simulink model "Linearization"  (R2022a)
settings: Solver=VariableStepAuto  StartTime=0.0  StopTime=100  RelTol=1e-3
undefined symbols (not defined in the file): Aactuator, ac, AeroCoeff, ControlAllocation, DUmax, DUmin, EngineTable, F, fcs, ft, g, hground, IC, kg, LandingGear, Light, LPmethod, m, MIL, Mode_deflection_aileron, Mode_deflection_elevator, Mode_deflection_rudder, Mode_deflection_TVC_y, Mode_deflection_TVC_z, N, Ninv_2nozzle, Ninv_no_nozzle, PIController, s, Sensor, slug, state0, sysID_DAQ, sysID_OBES, Umax_2nozzle, Umax_no_nozzle, Umin_2nozzle, Umin_no_nozzle, WMM2020
libraries: aerolibconvert2 x19, slpidlib x6, simulink x6, sharedutil x4, aerolibatmos2 x3, aerolibwind2 x3, aerolibbdyn x3, aerolibgravity2 x2, sharedtransform x1
(part 7 of 9)

== system Linearization/pqr NDI Controller/control matrix g1/Yawing  ==
  note: 註：因為 $\delta$ 單位是度(degree)，所以需要額外用 ${\left(\frac{\pi }{180°}\right)}$ 做單位換算
  note: $g_{r_{\delta_{rz} } } =\frac{-I_x l_T }{I_x I_z -I_{xz}^2 }\frac{T}{2}∙{\left(\frac{\pi }{180°}\right)}$
  note: 有指定port dimensions=[1,9]
  note: 1  gp_dra1
      | 2  gp_dla1
      | 3  gp_dre1
      | 4  gp_dle1
      | 5  gp_dr1
      | 6  gp_dra2
      | 7  gp_dla2
      | 8  gp_dre2
      | 9  gp_dle2
      | 10 gp_dr2
      |
      | 11 gq_dra
      | 12 gq_dla
      | 13 gq_dre
      | 14 gq_dle
      |
      | 15 gr_dra1
      | 16  gr_dla1
      | 17  gr_dre1
      | 18  gr_dle1
      | 19  gr_dr1
      | 20  gr_dra2
      | 21  gr_dla2
      | 22  gr_dre2
      | 23  gr_dle2
      | 24  gr_dr2
  note: 32 T/2
  note: 33 lt1
  note: 34 mt
  note: $g_{p_{\delta_r } } =\frac{1}{I_x I_z {-I}_{xz}^2 }{\left(I_{xz} \;∙\;g_{r_{\delta_{r1} } }+I_{x} \;∙\;g_{r_{\delta_{r2} } }\right)}$
  note: $g_{r_{\delta_{ra} } } =\frac{1}{I_x I_z {-I}_{xz}^2 }{\left\{I_{xz} \;∙\;g_{r_{\delta_{ra1} } }+I_{x} \;∙\;g_{r_{\delta_{ra2} } }\right\}}$
  note: $g_{r_{\delta_{re} } } =\frac{1}{I_x I_z {-I}_{xz}^2 }{\left\{I_{xz} \;∙\;g_{r_{\delta_{re1} } }+I_{x} \;∙\;g_{r_{\delta_{re2} } }\right\}}$
  note: $g_{r_{\delta_{le} } } =\frac{1}{I_x I_z {-I}_{xz}^2 }{\left\{I_{xz} \;∙\;g_{r_{\delta_{le1} } }+I_{x} \;∙\;g_{r_{\delta_{le2} } }\right\}}$
  note: $g_{r_{\delta_{la} } } =\frac{1}{I_x I_z {-I}_{xz}^2 }{\left\{I_{xz} \;∙\;g_{r_{\delta_{la1} } }+I_{x} \;∙\;g_{r_{\delta_{la2} } }\right\}}$
  note: $=-\begin{array}{l} \overset{-}{q} Sb{\left\{{\left(\frac{{\left[\Delta C_{n_{\delta_a } } +\Delta C_{n_{{\delta_a }_{LEF} } } ∙{\left(1-\frac{\delta_{LEF} }{25°}\right)}\right]}}{2}-\frac{{\left[\Delta C_{Y_{\delta_a } } +\Delta C_{Y_{{\delta_a }_{LEF} } } ∙{\left(1-\frac{\delta_{LEF} }{25°}\right)}\right]}}{2}∙{\left(x_{cg,ref} -x_{cg} \right)}∙\frac{\overset{-}{C} }{b}\right\}}\right)} \end{array}∙{\left(\frac{1}{20°}\right)}$
  note: $g_{r_{\delta_{r 2}} } =g_{p_{\delta_{r2} }$
  note: $=\begin{array}{l} -\overset{-}{q} Sb{\left\{{\left(C_{n_{\delta_{le} } } -{\left(x_{cg,ref} -x_{cg} \right)}∙\frac{\overset{-}{C} }{b}∙\Delta C_{Y_{\delta_e } } \right\}}\right)} \end{array}∙{\left(\frac{1}{25°}\right)}$
  note: $=\begin{array}{l} \overset{-}{q} Sb{\left\{{\left(\frac{{\left[\Delta C_{n_{\delta_a } } +\Delta C_{n_{{\delta_a }_{LEF} } } ∙{\left(1-\frac{\delta_{LEF} }{25°}\right)}\right]}}{2}-\frac{{\left[\Delta C_{Y_{\delta_a } } +\Delta C_{Y_{{\delta_a }_{LEF} } } ∙{\left(1-\frac{\delta_{LEF} }{25°}\right)}\right]}}{2}∙{\left(x_{cg,ref} -x_{cg} \right)}∙\frac{\overset{-}{C} }{b}\right\}}\right)} \end{array}∙{\left(\frac{1}{20°}\right)}$
  note: $=\bar{q} Sb∙{\left[\Delta C_{n_{\delta_r } } -{\left(x_{cg,ref} -x_{cg} \right)}∙\frac{\bar{c} }{b}∙\Delta C_{Y_{\delta_r } } \right]}∙{\left(\frac{1}{30°}\right)}$
  note: $g_{r_{\delta_{le2} } } =g_{p_{\delta_{le2} } }$
  note: $g_{r_{\delta_{ra2} } } =g_{p_{\delta_{ra2} } }$
  note: $g_{r_{\delta_{re2} } } =g_{p_{\delta_{re2} } }$
  note: $g_{r_{\delta_{la2} } } =g_{p_{\delta_{la2} } }$
  note: $=\begin{array}{l} \overset{-}{q} Sb{\left\{{\left(C_{n_{\delta_{re} } } -{\left(x_{cg,ref} -x_{cg} \right)}∙\frac{\overset{-}{C} }{b}∙\Delta C_{Y_{\delta_e } } \right\}}\right)} \end{array}∙{\left(\frac{1}{25°}\right)}$
  note: $g_{r_{\delta_{la1} } } =g_{p_{\delta_{la1} } }$
  note: $g_{r_{\delta_{le1} } }=g_{p_{\delta_{le1} } }$
  note: $g_{r_{\delta_{ra1} } } =g_{p_{\delta_{ra1} } }$
  note: $g_{r_{\delta_{re1} } } =g_{p_{\delta_{re1} } }$
  note: $=\begin{array}{l} -\overset{-}{q} Sb{\left\{{\left(C_{l_{\delta_{le} } } \right\}}\right)} \end{array}∙{\left(\frac{1}{25°}\right)}$
  note: $g_{r_{\delta_r 1} } =g_{p_{\delta_r 1} }$
  note: $=-\begin{array}{l} \overset{-}{q} Sb{\left\{{\left(\frac{{\left[\Delta C_{l_{\delta_a } } +\Delta C_{l_{{\delta_a }_{LEF} } } ∙{\left(1-\frac{\delta_{LEF} }{25°}\right)}\right]}}{2}\right\}}\right)} \end{array}∙{\left(\frac{1}{20°}\right)}$
  note: $=\bar{q} Sb∙\Delta C_{l_{\delta_r } } ∙{\left(\frac{1}{30°}\right)}$
  note: $=\begin{array}{l} \overset{-}{q} Sb{\left\{{\left(C_{l_{\delta_{re} } } \right\}}\right)} \end{array}∙{\left(\frac{1}{25°}\right)}$
  note: $=\begin{array}{l} \overset{-}{q} Sb{\left\{{\left(\frac{{\left[\Delta C_{l_{\delta_a } } +\Delta C_{l_{{\delta_a }_{LEF} } } ∙{\left(1-\frac{\delta_{LEF} }{25°}\right)}\right]}}{2}\right\}}\right)} \end{array}∙{\left(\frac{1}{20°}\right)}$
  note: 25 m
      | 26 Ix
      | 27 Iy
      | 28 Iz
      | 29 Ixy
      | 30 Ixz
      | 31 Iyz
  note: $g_{r_{\delta_{ry} } } =\frac{-I_{xz} m_T }{I_x I_z -I_{xz}^2 }\frac{T}{2}∙{\left(\frac{\pi }{180°}\right)}$
  note: $g_{r_{\delta_{lz} } } =\frac{-I_x l_T }{I_x I_z -I_{xz}^2 }\frac{T}{2}∙{\left(\frac{\pi }{180°}\right)}$
  note: $g_{r_{\delta_{ly} } } =\frac{I_{xz} m_T }{I_x I_z -I_{xz}^2 }\frac{T}{2}∙{\left(\frac{\pi }{180°}\right)}$
  note: $g_1 {\left({\overset{-}{x} }_1 \right)}={\left[\begin{array}{ccccccccc} g_{p_{\delta_{ra} } } & g_{p_{\delta_{la} } } & g_{p_{\delta_{re} } } & g_{p_{\delta_{le} } } & g_{p_{\delta_r } } & g_{p_{\delta_{ry} } } & g_{p_{\delta_{rz} } } & g_{p_{\delta_{ly} } } & g_{p_{\delta_{lz} } } \\ g_{q_{\delta_{ra} } } & g_{q_{\delta_{la} } } & g_{q_{\delta_{re} } } & g_{q_{\delta_{le} } } & 0 & g_{q_{\delta_{ry} } } & 0 & g_{q_{\delta_{ly} } } & 0 \\ g_{r_{\delta_{ra} } } & g_{r_{\delta_{la} } } & g_{r_{\delta_{re} } } & g_{r_{\delta_{le} } } & g_{r_{\delta_r } } & g_{r_{\delta_{ry} } } & g_{r_{\delta_{rz} } } & g_{r_{\delta_{ly} } } & g_{r_{\delta_{lz} } } \end{array}\right]}$
  control_g : Inport
  inertia : Inport  Port=2
  Thrust : Inport  Port=3
  "lt1 " : Inport  Port=4
  mt : Inport  Port=5
  Mux : Mux  Inputs=5
  Mux1 : Mux  Inputs=9
  yaw with TVC_lY : Fcn  Expr="(  u(30)*u(32)*u(34)  ) / ( u(26)*u(28)-u(30)^2 ) *pi/180"
  yaw with TVC_lZ : Fcn  Expr="(  -1*u(26)*u(32)*u(33)  ) / ( u(26)*u(28)-u(30)^2 ) *pi/180"
  yaw with TVC_rY : Fcn  Expr="(  -1*u(30)*u(32)*u(34)  ) / ( u(26)*u(28)-u(30)^2 ) *pi/180"
  yaw with TVC_rZ : Fcn  Expr="(  -1*u(26)*u(32)*u(33)  ) / ( u(26)*u(28)-u(30)^2 ) *pi/180"
  yaw with left aileron : Fcn  Expr=( ( u(30)*u(16)+u(26)*u(21) ) / ( u(26)*u(28)-u(30)^2 ) )
  yaw with left elevator : Fcn  Expr=( ( u(30)*u(18)+u(26)*u(23) ) / ( u(26)*u(28)-u(30)^2 ) )
  yaw with right aileron : Fcn  Expr=( ( u(30)*u(15)+u(26)*u(20) ) / ( u(26)*u(28)-u(30)^2 ) )
  yaw with right elevator : Fcn  Expr=( ( u(30)*u(17)+u(26)*u(22) ) / ( u(26)*u(28)-u(30)^2 ) )
  yaw with rudder : Fcn  Expr=( ( u(30)*u(19)+u(26)*u(24) ) / ( u(26)*u(28)-u(30)^2 ) )
  g1 Row3 : Outport  PortDimensions=[1,9]  VectorParamsAs1DForOutWhenUnconnected=off
  wires:
  control_g/1 -> Mux/1
  Mux1/1 -> g1 Row3/1
  inertia/1 -> Mux/2
  Thrust/1 -> Mux/3
  yaw with right aileron/1 -> Mux1/1
  "lt1 "/1 -> Mux/4
  Mux/1 -> yaw with TVC_rY/1, yaw with TVC_rZ/1, yaw with TVC_lZ/1, yaw with TVC_lY/1, yaw with rudder/1, yaw with left aileron/1, yaw with right aileron/1, yaw with right elevator/1, yaw with left elevator/1
  yaw with left aileron/1 -> Mux1/2
  yaw with right elevator/1 -> Mux1/3
  yaw with left elevator/1 -> Mux1/4
  yaw with rudder/1 -> Mux1/5
  yaw with TVC_rY/1 -> Mux1/6
  yaw with TVC_rZ/1 -> Mux1/7
  yaw with TVC_lY/1 -> Mux1/8
  yaw with TVC_lZ/1 -> Mux1/9
  mt/1 -> Mux/5

== system Linearization/sysID_Onboard_Excitation_System/signal generator/Pause Counter ==
  note: "Output when disabled" 設成 reset
      | 且 "Initial output" 設成 1
      | 目的是為了當 Enable = 0 時，令計數器重設為輸出 1
  note: "States when enabling" 設成 reset
      | 目的是為了當 Enable = 0 時，能將計數器重設成為1
  note: Pause Counter
  note: 內部有設定：
      | 1. sysID_OBES.Ts
      | 2. 計數器的初始值
  note: 計數器的累加值
  note: 具有暫停計數功能的計數器
  note: 允許計數的最大值
  note: 計數到最大值時，就暫停計數(+0)；
      | 否則，就繼續計數
  note: 參考資料： https://www.youtube.com/watch?v=utj-NZ5Hb6U
      | How to Design a Counter (Up/Down/Reset/Pause) in Simulink/MATLAB
  Enable : EnablePort  StatesWhenEnabling=reset
  Add : Sum
  Constant : Constant  Value=sysID_OBES.TVC_ry.size
  Constant2 : Constant  Value=0
  Constant3 : Constant
  Relational Operator : RelationalOperator  Operator===  OutDataTypeStr=boolean  RndMeth=Simplest  InputSameDT=off
  Switch : Switch  Criteria=u2 ~= 0  SaturateOnIntegerOverflow=off  InputSameDT=off
  Unit Delay : UnitDelay  SampleTime=sysID_OBES.Ts  HasFrameUpgradeWarning=on
  CountValue : Outport  OutputWhenDisabled=reset  InitialOutput=1
  isCountDone : Outport  Port=2
  wires:
  Add/1 -> CountValue/1, Unit Delay/1
  Relational Operator/1 -> isCountDone/1, Switch/2
  Constant/1 -> Relational Operator/1
  Unit Delay/1 -> Add/2, Relational Operator/2
  Switch/1 -> Add/1
  Constant2/1 -> Switch/1
  Constant3/1 -> Switch/3

== system Linearization/sysID_Onboard_Excitation_System/signal generator1/Pause Counter ==
  note: "Output when disabled" 設成 reset
      | 且 "Initial output" 設成 1
      | 目的是為了當 Enable = 0 時，令計數器重設為輸出 1
  note: "States when enabling" 設成 reset
      | 目的是為了當 Enable = 0 時，能將計數器重設成為1
  note: Pause Counter
  note: 內部有設定：
      | 1. sysID_OBES.Ts
      | 2. 計數器的初始值
  note: 計數器的累加值
  note: 具有暫停計數功能的計數器
  note: 允許計數的最大值
  note: 計數到最大值時，就暫停計數(+0)；
      | 否則，就繼續計數
  note: 參考資料： https://www.youtube.com/watch?v=utj-NZ5Hb6U
      | How to Design a Counter (Up/Down/Reset/Pause) in Simulink/MATLAB
  Enable : EnablePort  StatesWhenEnabling=reset
  Add : Sum
  Constant : Constant  Value=sysID_OBES.TVC_rz.size
  Constant2 : Constant  Value=0
  Constant3 : Constant
  Relational Operator : RelationalOperator  Operator===  OutDataTypeStr=boolean  RndMeth=Simplest  InputSameDT=off
  Switch : Switch  Criteria=u2 ~= 0  SaturateOnIntegerOverflow=off  InputSameDT=off
  Unit Delay : UnitDelay  SampleTime=sysID_OBES.Ts  HasFrameUpgradeWarning=on
  CountValue : Outport  OutputWhenDisabled=reset  InitialOutput=1
  isCountDone : Outport  Port=2
  wires:
  Add/1 -> CountValue/1, Unit Delay/1
  Relational Operator/1 -> isCountDone/1, Switch/2
  Constant/1 -> Relational Operator/1
  Unit Delay/1 -> Add/2, Relational Operator/2
  Switch/1 -> Add/1
  Constant2/1 -> Switch/1
  Constant3/1 -> Switch/3

== system Linearization/sysID_Onboard_Excitation_System/signal generator2/Pause Counter ==
  note: "Output when disabled" 設成 reset
      | 且 "Initial output" 設成 1
      | 目的是為了當 Enable = 0 時，令計數器重設為輸出 1
  note: "States when enabling" 設成 reset
      | 目的是為了當 Enable = 0 時，能將計數器重設成為1
  note: Pause Counter
  note: 內部有設定：
      | 1. sysID_OBES.Ts
      | 2. 計數器的初始值
  note: 計數器的累加值
  note: 具有暫停計數功能的計數器
  note: 允許計數的最大值
  note: 計數到最大值時，就暫停計數(+0)；
      | 否則，就繼續計數
  note: 參考資料： https://www.youtube.com/watch?v=utj-NZ5Hb6U
      | How to Design a Counter (Up/Down/Reset/Pause) in Simulink/MATLAB
  Enable : EnablePort  StatesWhenEnabling=reset
  Add : Sum
  Constant : Constant  Value=sysID_OBES.TVC_ly.size
  Constant2 : Constant  Value=0
  Constant3 : Constant
  Relational Operator : RelationalOperator  Operator===  OutDataTypeStr=boolean  RndMeth=Simplest  InputSameDT=off
  Switch : Switch  Criteria=u2 ~= 0  SaturateOnIntegerOverflow=off  InputSameDT=off
  Unit Delay : UnitDelay  SampleTime=sysID_OBES.Ts  HasFrameUpgradeWarning=on
  CountValue : Outport  OutputWhenDisabled=reset  InitialOutput=1
  isCountDone : Outport  Port=2
  wires:
  Add/1 -> CountValue/1, Unit Delay/1
  Relational Operator/1 -> isCountDone/1, Switch/2
  Constant/1 -> Relational Operator/1
  Unit Delay/1 -> Add/2, Relational Operator/2
  Switch/1 -> Add/1
  Constant2/1 -> Switch/1
  Constant3/1 -> Switch/3

== system Linearization/sysID_Onboard_Excitation_System/signal generator3/Pause Counter ==
  note: "Output when disabled" 設成 reset
      | 且 "Initial output" 設成 1
      | 目的是為了當 Enable = 0 時，令計數器重設為輸出 1
  note: "States when enabling" 設成 reset
      | 目的是為了當 Enable = 0 時，能將計數器重設成為1
  note: Pause Counter
  note: 內部有設定：
      | 1. sysID_OBES.Ts
      | 2. 計數器的初始值
  note: 計數器的累加值
  note: 具有暫停計數功能的計數器
  note: 允許計數的最大值
  note: 計數到最大值時，就暫停計數(+0)；
      | 否則，就繼續計數
  note: 參考資料： https://www.youtube.com/watch?v=utj-NZ5Hb6U
      | How to Design a Counter (Up/Down/Reset/Pause) in Simulink/MATLAB
  Enable : EnablePort  StatesWhenEnabling=reset
  Add : Sum
  Constant : Constant  Value=sysID_OBES.TVC_lz.size
  Constant2 : Constant  Value=0
  Constant3 : Constant
  Relational Operator : RelationalOperator  Operator===  OutDataTypeStr=boolean  RndMeth=Simplest  InputSameDT=off
  Switch : Switch  Criteria=u2 ~= 0  SaturateOnIntegerOverflow=off  InputSameDT=off
  Unit Delay : UnitDelay  SampleTime=sysID_OBES.Ts  HasFrameUpgradeWarning=on
  CountValue : Outport  OutputWhenDisabled=reset  InitialOutput=1
  isCountDone : Outport  Port=2
  wires:
  Add/1 -> CountValue/1, Unit Delay/1
  Relational Operator/1 -> isCountDone/1, Switch/2
  Constant/1 -> Relational Operator/1
  Unit Delay/1 -> Add/2, Relational Operator/2
  Switch/1 -> Add/1
  Constant2/1 -> Switch/1
  Constant3/1 -> Switch/3

== system Linearization/sysID_Onboard_Excitation_System/signal generator4/Pause Counter ==
  note: "Output when disabled" 設成 reset
      | 且 "Initial output" 設成 1
      | 目的是為了當 Enable = 0 時，令計數器重設為輸出 1
  note: "States when enabling" 設成 reset
      | 目的是為了當 Enable = 0 時，能將計數器重設成為1
  note: Pause Counter
  note: 內部有設定：
      | 1. sysID_OBES.Ts
      | 2. 計數器的初始值
  note: 計數器的累加值
  note: 具有暫停計數功能的計數器
  note: 允許計數的最大值
  note: 計數到最大值時，就暫停計數(+0)；
      | 否則，就繼續計數
  note: 參考資料： https://www.youtube.com/watch?v=utj-NZ5Hb6U
      | How to Design a Counter (Up/Down/Reset/Pause) in Simulink/MATLAB
  Enable : EnablePort  StatesWhenEnabling=reset
  Add : Sum
  Constant : Constant  Value=sysID_OBES.right_aileron.size
  Constant2 : Constant  Value=0
  Constant3 : Constant
  Relational Operator : RelationalOperator  Operator===  OutDataTypeStr=boolean  RndMeth=Simplest  InputSameDT=off
  Switch : Switch  Criteria=u2 ~= 0  SaturateOnIntegerOverflow=off  InputSameDT=off
  Unit Delay : UnitDelay  SampleTime=sysID_OBES.Ts  HasFrameUpgradeWarning=on
  CountValue : Outport  OutputWhenDisabled=reset  InitialOutput=1
  isCountDone : Outport  Port=2
  wires:
  Add/1 -> CountValue/1, Unit Delay/1
  Relational Operator/1 -> isCountDone/1, Switch/2
  Constant/1 -> Relational Operator/1
  Unit Delay/1 -> Add/2, Relational Operator/2
  Switch/1 -> Add/1
  Constant2/1 -> Switch/1
  Constant3/1 -> Switch/3

== system Linearization/sysID_Onboard_Excitation_System/signal generator5/Pause Counter ==
  note: "Output when disabled" 設成 reset
      | 且 "Initial output" 設成 1
      | 目的是為了當 Enable = 0 時，令計數器重設為輸出 1
  note: "States when enabling" 設成 reset
      | 目的是為了當 Enable = 0 時，能將計數器重設成為1
  note: Pause Counter
  note: 內部有設定：
      | 1. sysID_OBES.Ts
      | 2. 計數器的初始值
  note: 計數器的累加值
  note: 具有暫停計數功能的計數器
  note: 允許計數的最大值
  note: 計數到最大值時，就暫停計數(+0)；
      | 否則，就繼續計數
  note: 參考資料： https://www.youtube.com/watch?v=utj-NZ5Hb6U
      | How to Design a Counter (Up/Down/Reset/Pause) in Simulink/MATLAB
  Enable : EnablePort  StatesWhenEnabling=reset
  Add : Sum
  Constant : Constant  Value=sysID_OBES.left_aileron.size
  Constant2 : Constant  Value=0
  Constant3 : Constant
  Relational Operator : RelationalOperator  Operator===  OutDataTypeStr=boolean  RndMeth=Simplest  InputSameDT=off
  Switch : Switch  Criteria=u2 ~= 0  SaturateOnIntegerOverflow=off  InputSameDT=off
  Unit Delay : UnitDelay  SampleTime=sysID_OBES.Ts  HasFrameUpgradeWarning=on
  CountValue : Outport  OutputWhenDisabled=reset  InitialOutput=1
  isCountDone : Outport  Port=2
  wires:
  Add/1 -> CountValue/1, Unit Delay/1
  Relational Operator/1 -> isCountDone/1, Switch/2
  Constant/1 -> Relational Operator/1
  Unit Delay/1 -> Add/2, Relational Operator/2
  Switch/1 -> Add/1
  Constant2/1 -> Switch/1
  Constant3/1 -> Switch/3

== system Linearization/sysID_Onboard_Excitation_System/signal generator6/Pause Counter ==
  note: "Output when disabled" 設成 reset
      | 且 "Initial output" 設成 1
      | 目的是為了當 Enable = 0 時，令計數器重設為輸出 1
  note: "States when enabling" 設成 reset
      | 目的是為了當 Enable = 0 時，能將計數器重設成為1
  note: Pause Counter
  note: 內部有設定：
      | 1. sysID_OBES.Ts
      | 2. 計數器的初始值
  note: 計數器的累加值
  note: 具有暫停計數功能的計數器
  note: 允許計數的最大值
  note: 計數到最大值時，就暫停計數(+0)；
      | 否則，就繼續計數
  note: 參考資料： https://www.youtube.com/watch?v=utj-NZ5Hb6U
      | How to Design a Counter (Up/Down/Reset/Pause) in Simulink/MATLAB
  Enable : EnablePort  StatesWhenEnabling=reset
  Add : Sum
  Constant : Constant  Value=sysID_OBES.right_elevator.size
  Constant2 : Constant  Value=0
  Constant3 : Constant
  Relational Operator : RelationalOperator  Operator===  OutDataTypeStr=boolean  RndMeth=Simplest  InputSameDT=off
  Switch : Switch  Criteria=u2 ~= 0  SaturateOnIntegerOverflow=off  InputSameDT=off
  Unit Delay : UnitDelay  SampleTime=sysID_OBES.Ts  HasFrameUpgradeWarning=on
  CountValue : Outport  OutputWhenDisabled=reset  InitialOutput=1
  isCountDone : Outport  Port=2
  wires:
  Add/1 -> CountValue/1, Unit Delay/1
  Relational Operator/1 -> isCountDone/1, Switch/2
  Constant/1 -> Relational Operator/1
  Unit Delay/1 -> Add/2, Relational Operator/2
  Switch/1 -> Add/1
  Constant2/1 -> Switch/1
  Constant3/1 -> Switch/3

== system Linearization/sysID_Onboard_Excitation_System/signal generator7/Pause Counter ==
  note: "Output when disabled" 設成 reset
      | 且 "Initial output" 設成 1
      | 目的是為了當 Enable = 0 時，令計數器重設為輸出 1
  note: "States when enabling" 設成 reset
      | 目的是為了當 Enable = 0 時，能將計數器重設成為1
  note: Pause Counter
  note: 內部有設定：
      | 1. sysID_OBES.Ts
      | 2. 計數器的初始值
  note: 計數器的累加值
  note: 具有暫停計數功能的計數器
  note: 允許計數的最大值
  note: 計數到最大值時，就暫停計數(+0)；
      | 否則，就繼續計數
  note: 參考資料： https://www.youtube.com/watch?v=utj-NZ5Hb6U
      | How to Design a Counter (Up/Down/Reset/Pause) in Simulink/MATLAB
  Enable : EnablePort  StatesWhenEnabling=reset
  Add : Sum
  Constant : Constant  Value=sysID_OBES.left_elevator.size
  Constant2 : Constant  Value=0
  Constant3 : Constant
  Relational Operator : RelationalOperator  Operator===  OutDataTypeStr=boolean  RndMeth=Simplest  InputSameDT=off
  Switch : Switch  Criteria=u2 ~= 0  SaturateOnIntegerOverflow=off  InputSameDT=off
  Unit Delay : UnitDelay  SampleTime=sysID_OBES.Ts  HasFrameUpgradeWarning=on
  CountValue : Outport  OutputWhenDisabled=reset  InitialOutput=1
  isCountDone : Outport  Port=2
  wires:
  Add/1 -> CountValue/1, Unit Delay/1
  Relational Operator/1 -> isCountDone/1, Switch/2
  Constant/1 -> Relational Operator/1
  Unit Delay/1 -> Add/2, Relational Operator/2
  Switch/1 -> Add/1
  Constant2/1 -> Switch/1
  Constant3/1 -> Switch/3

== system Linearization/sysID_Onboard_Excitation_System/signal generator8/Pause Counter ==
  note: "Output when disabled" 設成 reset
      | 且 "Initial output" 設成 1
      | 目的是為了當 Enable = 0 時，令計數器重設為輸出 1
  note: "States when enabling" 設成 reset
      | 目的是為了當 Enable = 0 時，能將計數器重設成為1
  note: Pause Counter
  note: 內部有設定：
      | 1. sysID_OBES.Ts
      | 2. 計數器的初始值
  note: 計數器的累加值
  note: 具有暫停計數功能的計數器
  note: 允許計數的最大值
  note: 計數到最大值時，就暫停計數(+0)；
      | 否則，就繼續計數
  note: 參考資料： https://www.youtube.com/watch?v=utj-NZ5Hb6U
      | How to Design a Counter (Up/Down/Reset/Pause) in Simulink/MATLAB
  Enable : EnablePort  StatesWhenEnabling=reset
  Add : Sum
  Constant : Constant  Value=sysID_OBES.rudder.size
  Constant2 : Constant  Value=0
  Constant3 : Constant
  Relational Operator : RelationalOperator  Operator===  OutDataTypeStr=boolean  RndMeth=Simplest  InputSameDT=off
  Switch : Switch  Criteria=u2 ~= 0  SaturateOnIntegerOverflow=off  InputSameDT=off
  Unit Delay : UnitDelay  SampleTime=sysID_OBES.Ts  HasFrameUpgradeWarning=on
  CountValue : Outport  OutputWhenDisabled=reset  InitialOutput=1
  isCountDone : Outport  Port=2
  wires:
  Add/1 -> CountValue/1, Unit Delay/1
  Relational Operator/1 -> isCountDone/1, Switch/2
  Constant/1 -> Relational Operator/1
  Unit Delay/1 -> Add/2, Relational Operator/2
  Switch/1 -> Add/1
  Constant2/1 -> Switch/1
  Constant3/1 -> Switch/3

== system Linearization/Vehicle/6DOF (Quaternion)/Accerlation_offset/accerlation_x ==
  ax_cg : Inport
  q : Inport  Port=2
  r : Inport  Port=3
  position_x : Inport  Port=4
  p : Inport  Port=5
  r_dot : Inport  Port=6
  position_y : Inport  Port=7
  q_dot : Inport  Port=8
  position_z : Inport  Port=9
  ax_bias : Inport  Port=10
  Add3 : Sum
  Add4 : Sum
  Math Function : Math  Operator=square
  Math Function1 : Math  Operator=square
  Product{,1..4} (5 alike) : Product
  Subtract : Sum  Inputs=+-+++
  Subtract1 : Sum  Inputs=+-
  ax_as : Outport
  wires:
  Math Function1/1 -> Add3/2
  Product1/1 -> Subtract1/1
  Add4/1 -> Product4/1
  Product3/1 -> Add4/1
  Subtract1/1 -> Product2/1
  Math Function/1 -> Add3/1
  r_dot/1 -> Subtract1/2
  Product2/1 -> Subtract/3
  Add3/1 -> Product/1
  position_x/1 -> Product/2
  Product4/1 -> Subtract/4
  Product/1 -> Subtract/2
  ax_bias/1 -> Subtract/5
  r/1 -> Product3/2, Math Function1/1
  position_z/1 -> Product4/2
  q/1 -> Product1/2, Math Function/1
  Subtract/1 -> ax_as/1
  p/1 -> Product3/1, Product1/1
  q_dot/1 -> Add4/2
  ax_cg/1 -> Subtract/1
  position_y/1 -> Product2/2

== system Linearization/Vehicle/6DOF (Quaternion)/Accerlation_offset/accerlation_y ==
  ay_cg : Inport
  p : Inport  Port=2
  r : Inport  Port=3
  position_y : Inport  Port=4
  q : Inport  Port=5
  p_dot : Inport  Port=6
  position_z : Inport  Port=7
  r_dot : Inport  Port=8
  position_x : Inport  Port=9
  ay_bias : Inport  Port=10
  Math Function2 : Math  Operator=square
  Math Function3 : Math  Operator=square
  Product{5..9} (5 alike) : Product
  Subtract2 : Sum
  Subtract3 : Sum
  Subtract5 : Sum  Inputs=+-
  Subtract6 : Sum  Inputs=+-+++
  ay_as : Outport
  wires:
  Product5/1 -> Subtract6/2
  Product9/1 -> Subtract6/4
  ay_bias/1 -> Subtract6/5
  Subtract3/1 -> Product9/1
  Subtract6/1 -> ay_as/1
  Subtract5/1 -> Product7/1
  q/1 -> Product8/2, Product6/1
  Subtract2/1 -> Product5/1
  Product7/1 -> Subtract6/3
  Product8/1 -> Subtract3/1
  Math Function3/1 -> Subtract2/2
  Product6/1 -> Subtract5/1
  position_x/1 -> Product9/2
  Math Function2/1 -> Subtract2/1
  r/1 -> Product6/2, Math Function3/1
  ay_cg/1 -> Subtract6/1
  position_y/1 -> Product5/2
  r_dot/1 -> Subtract3/2
  p/1 -> Math Function2/1, Product8/1
  position_z/1 -> Product7/2
  p_dot/1 -> Subtract5/2

== system Linearization/Vehicle/6DOF (Quaternion)/Accerlation_offset/accerlation_z ==
  az_cg : Inport
  p : Inport  Port=2
  q : Inport  Port=3
  position_z : Inport  Port=4
  r : Inport  Port=5
  q_dot : Inport  Port=6
  position_x : Inport  Port=7
  p_dot : Inport  Port=8
  position_y : Inport  Port=9
  az_bias : Inport  Port=10
  Math Function4 : Math  Operator=square
  Math Function5 : Math  Operator=square
  Product{10..14} (5 alike) : Product
  Subtract4 : Sum
  Subtract7 : Sum
  Subtract8 : Sum  Inputs=+-+++
  Subtract9 : Sum  Inputs=+-
  az_as : Outport
  wires:
  Math Function5/1 -> Subtract4/2
  Math Function4/1 -> Subtract4/1
  Subtract4/1 -> Product10/1
  Subtract7/1 -> Product14/1
  q/1 -> Product13/1, Math Function5/1
  Product12/1 -> Subtract8/3
  Product14/1 -> Subtract8/4
  Product13/1 -> Subtract7/1
  Product11/1 -> Subtract9/1
  position_y/1 -> Product14/2
  Subtract9/1 -> Product12/1
  Product10/1 -> Subtract8/2
  az_cg/1 -> Subtract8/1
  q_dot/1 -> Subtract9/2
  az_bias/1 -> Subtract8/5
  p_dot/1 -> Subtract7/2
  r/1 -> Product13/2, Product11/2
  position_x/1 -> Product12/2
  Subtract8/1 -> az_as/1
  p/1 -> Product11/1, Math Function4/1
  position_z/1 -> Product10/2

== system Linearization/Vehicle/Actuators (no roll off)1/Engine block/If Action Subsystem ==
  note: Pow_max
      |
      | Pow_min
      |
      | T_idle
      |
      | T_mil
      |
      | T_max
  "input " : Inport
  Action Port : ActionPort
  Add : Sum
  Add1 : Sum  Inputs=-+
  Demux : Demux  Outputs=5
  Divide : Product  Inputs=**
  Gain : Gain  Gain=1/50
  Terminator : Terminator
  Terminator1 : Terminator
  T_max1 : Outport  VectorParamsAs1DForOutWhenUnconnected=off
  wires:
  Demux/3 -> Add1/1, Add/1
  Demux/4 -> Add1/2
  Add1/1 -> Divide/2
  Gain/1 -> Divide/1
  Divide/1 -> Add/2
  Add/1 -> T_max1/1
  "input "/1 -> Demux/1
  Demux/1 -> Gain/1
  Demux/2 -> Terminator/1
  Demux/5 -> Terminator1/1

== system Linearization/Vehicle/Actuators (no roll off)1/Engine block/If Action Subsystem1 ==
  note: Pow_max
      |
      | Pow_min
      |
      | T_idle
      |
      | T_mil
      |
      | T_max
  "input " : Inport
  Action Port : ActionPort
  Add : Sum
  Add1 : Sum  Inputs=-+
  Add2 : Sum  Inputs=-+
  Constant : Constant  Value=50
  Demux : Demux  Outputs=5
  Gain : Gain  Gain=1/50
  Product : Product
  Terminator : Terminator
  Terminator1 : Terminator
  T_max1 : Outport  VectorParamsAs1DForOutWhenUnconnected=off
  wires:
  "input "/1 -> Demux/1
  Demux/4 -> Add/2, Add1/1
  Demux/5 -> Add1/2
  Demux/1 -> Add2/2
  Constant/1 -> Add2/1
  Add2/1 -> Gain/1
  Add1/1 -> Product/2
  Gain/1 -> Product/1
  Product/1 -> Add/1
  Add/1 -> T_max1/1
  Demux/3 -> Terminator1/1
  Demux/2 -> Terminator/1

== system Linearization/Vehicle/Actuators (no roll off)1/Engine block/If Action Subsystem2 ==
  note: Pow_max
      |
      | Pow_min
      |
      | T_idle
      |
      | T_mil
      |
      | T_max
  "input " : Inport
  Action Port : ActionPort
  Add : Sum
  Add1 : Sum  Inputs=-+
  Demux : Demux  Outputs=5
  Divide : Product  Inputs=**
  Gain : Gain  Gain=1/50
  Terminator : Terminator
  Terminator1 : Terminator
  T_min : Outport  VectorParamsAs1DForOutWhenUnconnected=off
  wires:
  Demux/3 -> Add1/1, Add/1
  Demux/4 -> Add1/2
  Add1/1 -> Divide/2
  Gain/1 -> Divide/1
  Divide/1 -> Add/2
  Add/1 -> T_min/1
  "input "/1 -> Demux/1
  Demux/2 -> Gain/1
  Demux/5 -> Terminator1/1
  Demux/1 -> Terminator/1

== system Linearization/Vehicle/Actuators (no roll off)1/Engine block/If Action Subsystem3 ==
  note: Pow_max
      |
      | Pow_min
      |
      | T_idle
      |
      | T_mil
      |
      | T_max
  "input " : Inport
  Action Port : ActionPort
  Add : Sum
  Add1 : Sum  Inputs=-+
  Add2 : Sum  Inputs=-+
  Constant : Constant  Value=50
  Demux : Demux  Outputs=5
  Gain : Gain  Gain=1/50
  Product : Product
  Terminator : Terminator
  Terminator1 : Terminator
  T_min : Outport  VectorParamsAs1DForOutWhenUnconnected=off
  wires:
  "input "/1 -> Demux/1
  Demux/4 -> Add/2, Add1/1
  Demux/5 -> Add1/2
  Constant/1 -> Add2/1
  Add2/1 -> Gain/1
  Add1/1 -> Product/2
  Gain/1 -> Product/1
  Product/1 -> Add/1
  Add/1 -> T_min/1
  Demux/3 -> Terminator1/1
  Demux/2 -> Add2/2
  Demux/1 -> Terminator/1

== system Linearization/Vehicle/Aerodynamics/Aerofynamic Coefficients/CXT ==
  note: 氣動力表格僅提供到攻角到
      | 45度，超過45度後皆採用45
      | 度的氣動力係數
  note: $C_{X,T} =C_X {\left(\alpha ,\beta ,\delta_e \right)}+\Delta C_{X_{LEF} } ∙{\left(1-\frac{\delta_{LEF} }{25°}\right)}+\frac{q\overset{-}{c} }{2V_T }∙{\left[C_{X_q } {\left(\alpha \right)}+\Delta C_{X_{q_{LEF} } } {\left(\alpha \right)}∙{\left(1-\frac{\delta_{LEF} }{25°}\right)}\right]}+\mathrm{\ }\Delta C_{X_{SB} } {\left(\alpha \right)}∙{\left(\frac{\delta_{SB} }{60°}\right)}+C_{X_{\delta_{ra} } } {∙\delta }_{ra} +C_{X_{\delta_{la} } } {∙\delta }_{la}$
  note: 體軸 x 方向之氣動力係數 (total x-axis force coefficient)：
  note: ${\hat{X} }_{\delta_e } =\frac{C_X {\left(\alpha ,\beta ,\delta_e +0.1\right)}-C_X {\left(\alpha ,\beta ,\delta_e -0.1\right)}}{0.2}$
  note: $C_{X_{\delta_{ra} } } =C_{X_{\delta la} } =\frac{{\hat{X} }_{\delta_e } }{2}∙0.4$
  note: $\Delta C_{X_{LEF} } =C_{X_{LEF} } {\left(\alpha ,\beta \right)}-C_X {\left(\alpha ,\beta ,\delta_e =0°\right)}$
  note: ${\hat{X} }_{\delta_e } =\frac{C_X {\left(\alpha ,\beta ,\delta_e +0.1\right)}-C_X {\left(\alpha ,\beta ,\delta_e -0.1\right)}}{0.2}$
  note: $C_{X_{\delta_{ra} } } =C_{X_{\delta la} } =\frac{{\hat{X} }_{\delta_e } }{2}∙0.4$
  alpha (deg) : Inport
  "beta (deg) " : Inport  Port=2
  right elevator (deg) : Inport  Port=3
  left elevator (deg) : Inport  Port=4
  dlef : Inport  Port=5
  qc_2v : Inport  Port=6
  sb : Inport  Port=7
  right aileron(rad) : Inport  Port=8
  left aileron(rad) : Inport  Port=9
  Add : Sum  Inputs=+-
  Add1 : Sum  Inputs=+++++
  Add{2..4,7} (4 alike) : Sum
  Add5 : Sum  Inputs=+-
  Add6 : Sum  Inputs=+-
  Constant : Constant  Value=0.1
  Constant1 : Constant  Value=0.1
  Constant2 : Constant  Value=0.2
  Cx : Interpolation_n-D  NumberOfTableDimensions=3  Table=AeroCoeff.Cx
      settings: InputPortMap=u0,u1,u2,u3,u4,u5
  Cx1 : Interpolation_n-D  NumberOfTableDimensions=3  Table=AeroCoeff.Cx
      settings: InputPortMap=u0,u1,u2,u3,u4,u5
  Cx2 : Interpolation_n-D  NumberOfTableDimensions=3  Table=AeroCoeff.Cx
      settings: InputPortMap=u0,u1,u2,u3,u4,u5
  Cx_elevator0 : Interpolation_n-D  Table=AeroCoeff.Cx_elevator0
  Cx_lef : Interpolation_n-D  Table=AeroCoeff.Cx_lef
  "Cx_q " : Interpolation_n-D  NumberOfTableDimensions=1  Table=AeroCoeff.Cx_q
      settings: InputPortMap=u0,u1
  Cx_q_lef : Interpolation_n-D  NumberOfTableDimensions=1  Table=AeroCoeff.Cx_q_lef
      settings: InputPortMap=u0,u1
  Divide : Product  Inputs=*/
  Gain : Gain  Gain=20
  Gain2 : Gain  Gain=(1/2)*0.4
  Gain3 : Gain  Gain=20
  Gain4 : Gain  Gain=1/2
  Product{,1..5} (6 alike) : Product
  alpha Prelookup : PreLookup  BreakpointsData=AeroCoeff.alpha_prelookup  IndexSearchMethod=Linear search  BeginIndexSearchUsingPreviousIndexResult=on  DiagnosticForOutOfRangeInput=Warning
  beta Prelookup : PreLookup  BreakpointsData=AeroCoeff.beta_prelookup  IndexSearchMethod=Linear search  BeginIndexSearchUsingPreviousIndexResult=on  DiagnosticForOutOfRangeInput=Warning
  dCX_sb : Interpolation_n-D  NumberOfTableDimensions=1  Table=AeroCoeff.dCX_sb
      settings: InputPortMap=u0,u1
  elevator Prelookup : PreLookup  BreakpointsData=AeroCoeff.elevator_prelookup2  IndexSearchMethod=Linear search  BeginIndexSearchUsingPreviousIndexResult=on  DiagnosticForOutOfRangeInput=Warning
  elevator Prelookup1 : PreLookup  BreakpointsData=AeroCoeff.elevator_prelookup2  IndexSearchMethod=Linear search  BeginIndexSearchUsingPreviousIndexResult=on  DiagnosticForOutOfRangeInput=Warning
  elevator Prelookup2 : PreLookup  BreakpointsData=AeroCoeff.elevator_prelookup2  IndexSearchMethod=Linear search  BeginIndexSearchUsingPreviousIndexResult=on  DiagnosticForOutOfRangeInput=Warning
  Cx_tot : Outport  VectorParamsAs1DForOutWhenUnconnected=off
  wires:
  beta Prelookup/2 -> Cx2/4, Cx1/4, Cx_elevator0/4, Cx_lef/4, Cx/4
  beta Prelookup/1 -> Cx2/3, Cx1/3, Cx_elevator0/3, Cx_lef/3, Cx/3
  Cx_lef/1 -> Add/1
  alpha Prelookup/1 -> Cx_q_lef/1, Cx2/1, Cx1/1, dCX_sb/1, "Cx_q "/1, Cx_elevator0/1, Cx/1, Cx_lef/1
  elevator Prelookup/2 -> Cx/6
  "beta (deg) "/1 -> beta Prelookup/1
  Add/1 -> Product/1
  alpha Prelookup/2 -> Cx_q_lef/2, Cx2/2, Cx1/2, dCX_sb/2, "Cx_q "/2, Cx_elevator0/2, Cx_lef/2, Cx/2
  Product/1 -> Add1/2
  elevator Prelookup/1 -> Cx/5
  Add2/1 -> Product2/1
  Cx/1 -> Add1/1
  Cx_elevator0/1 -> Add/2
  Cx_q_lef/1 -> Product1/1
  Product1/1 -> Add2/2
  "Cx_q "/1 -> Add2/1
  dlef/1 -> Product/2, Product1/2
  Product2/1 -> Add1/3
  Add1/1 -> Cx_tot/1
  qc_2v/1 -> Product2/2
  dCX_sb/1 -> Product3/1
  sb/1 -> Product3/2
  Product3/1 -> Add1/4
  alpha (deg)/1 -> alpha Prelookup/1
  Add3/1 -> Gain4/1
  right elevator (deg)/1 -> Add3/1
  left elevator (deg)/1 -> Add3/2
  Add4/1 -> elevator Prelookup1/1
  Constant/1 -> Add4/2
  Constant1/1 -> Add5/2
  Add5/1 -> elevator Prelookup2/1
  elevator Prelookup1/1 -> Cx1/5
  elevator Prelookup1/2 -> Cx1/6
  Cx1/1 -> Add6/1
  Cx2/1 -> Add6/2
  Add6/1 -> Divide/1
  Divide/1 -> Gain2/1
  right aileron(rad)/1 -> Gain/1
  Gain2/1 -> Product5/1, Product4/1
  left aileron(rad)/1 -> Gain3/1
  Product4/1 -> Add7/1
  Product5/1 -> Add7/2
  Add7/1 -> Add1/5
  Constant2/1 -> Divide/2
  Gain/1 -> Product4/2
  Gain3/1 -> Product5/2
  elevator Prelookup2/1 -> Cx2/5
  elevator Prelookup2/2 -> Cx2/6
  Gain4/1 -> Add4/1, Add5/1, elevator Prelookup/1

== system Linearization/Vehicle/Aerodynamics/Aerofynamic Coefficients/CYT ==
  note: $\Delta C_{Y_{\delta_a } }$
  note: 氣動力表格僅提供到攻角到
      | 45度，超過45度後皆採用45
      | 度的氣動力係數
  note: 氣動力表格僅提供到攻角到
      | 45度，超過45度後皆採用45
      | 度的氣動力係數
  note: 體軸 y 方向之氣動力係數 (total y-axis force coefficient)：
  note: $C_{Y_{\delta_{re} } } =C_{Y_{\delta_{le} } } =\frac{\Delta C_{Y_{\delta_a } } }{2}∙0.68$
  note: $C_{Y,T} \ \ \ =\ \ \ \ C_Y {\left(\alpha ,\beta \right)}+\Delta C_{Y_{LEF} } ∙{\left(1-\frac{\delta_{LEF} }{25°}\right)}+\frac{pb}{2V_T }∙{\left[C_{Y_p } {\left(\alpha \right)}+\Delta C_{{Y_p }_{LEF} } {\left(\alpha \right)}∙{\left(1-\frac{\delta_{LEF} }{25°}\right)}\right]}+\ \frac{rb}{2V_T }∙{\left[C_{Y_r } {\left(\alpha \right)}+\Delta C_{{Y_r }_{LEF} } {\left(\alpha \right)}∙{\left(1-\frac{\delta_{LEF} }{25°}\right)}\right]}+\Delta C_{Y_{\delta_r } } ∙{\left(\frac{\delta_r }{30°}\right)}+\frac{{\left[\Delta C_{Y_{\delta_a } } +\Delta C_{Y_{{\delta_a }_{LEF} } } ∙{\left(1-\frac{\delta_{LEF} }{25°}\right)}\right]}}{2}∙{\left(\frac{\delta_{ra} }{20°}\right)}-\frac{{\left[\Delta C_{Y_{\delta_a } } +\Delta C_{Y_{{\delta_a }_{LEF} } } ∙{\left(1-\frac{\delta_{LEF} }{25°}\right)}\right]}}{2}∙{\left(\frac{\delta_{la} }{20°}\right)}{+C}_{Y_{\delta_{re} } } ∙{\left(\frac{\delta_{re} }{25°}\right)}-C_{Y_{\delta_{le} } } ∙{\left(\frac{\delta_{le} }{25°}\right)}$
  note: $\Delta C_{Y_{\delta_r } }=C_{Y_{\delta_r =30°} } {\left(\alpha ,\beta \right)}-C_Y {\left(\alpha ,\beta \right)}$
  note: $\Delta C_{Y_{{\delta_a }_{LEF} } } =C_{Y_{{\delta_a =20°}_{LEF} } } {\left(\alpha ,\beta \right)}-C_{Y_{LEF} } {\left(\alpha ,\beta \right)}-\Delta C_{Y_{\delta_a } }$
  note: $\Delta C_{Y_{LEF} }=C_{Y_{LEF} } {\left(\alpha ,\beta \right)}\ \ -C_Y {\left(\alpha ,\beta \right)}$
  note: $\Delta C_{Y_{\delta_a } }=C_{Y_{\delta_a =20°} } {\left(\alpha ,\beta \right)}-C_Y {\left(\alpha ,\beta \right)}$
  note: $C_{Y_{\delta_{re} } } =C_{Y_{\delta_{le} } } =\frac{\Delta C_{Y_{\delta_a } } }{2}∙0.68$
  note: $\Delta C_{Y_{\delta_a } } =C_{Y_{\delta_a =20°} } {\left(\alpha ,\beta \right)}-C_Y {\left(\alpha ,\beta \right)}$
  alpha (deg) : Inport
  beta (deg) : Inport  Port=2
  dlef : Inport  Port=3
  right aileron(rad) : Inport  Port=4
  left aileron(rad) : Inport  Port=5
  drud : Inport  Port=6
  rb_2v : Inport  Port=7
  pb_2v : Inport  Port=8
  right elevator : Inport  Port=9
  left elevator : Inport  Port=10
  Add : Sum  Inputs=-+
  Add1 : Sum  Inputs=-+
  Add2 : Sum  Inputs=+--
  Add3 : Sum  Inputs=+-
  Add4 : Sum  Inputs=+++++++
  Add5 : Sum
  Add6 : Sum
  Add7 : Sum
  Add8 : Sum  Inputs=+-
  Add9 : Sum  Inputs=+-
  CY : Interpolation_n-D  Table=AeroCoeff.CY
  CY_delta_ail : Interpolation_n-D  Table=AeroCoeff.CY_delta_ail
  CY_delta_ail_lef : Interpolation_n-D  Table=AeroCoeff.CY_delta_ail_lef
  CY_delta_r : Interpolation_n-D  Table=AeroCoeff.CY_delta_r
  CY_lef : Interpolation_n-D  Table=AeroCoeff.CY_lef
  CY_p : Interpolation_n-D  NumberOfTableDimensions=1  Table=AeroCoeff.CY_p
      settings: InputPortMap=u0,u1
  CY_r : Interpolation_n-D  NumberOfTableDimensions=1  Table=AeroCoeff.CY_r
      settings: InputPortMap=u0,u1
  Gain : Gain  Gain=1/2
  Gain1 : Gain  Gain=1/25
  Gain2 : Gain  Gain=(1/2)*0.68
  Product{,1..8} (9 alike) : Product
  alpha Prelookup : PreLookup  BreakpointsData=AeroCoeff.alpha_prelookup  IndexSearchMethod=Linear search  BeginIndexSearchUsingPreviousIndexResult=on  DiagnosticForOutOfRangeInput=Warning
  beta Prelookup : PreLookup  BreakpointsData=AeroCoeff.beta_prelookup  IndexSearchMethod=Linear search  BeginIndexSearchUsingPreviousIndexResult=on  DiagnosticForOutOfRangeInput=Warning
  dCY_p_lef : Interpolation_n-D  NumberOfTableDimensions=1  Table=AeroCoeff.dCY_p_lef
      settings: InputPortMap=u0,u1
  dCY_r_lef : Interpolation_n-D  NumberOfTableDimensions=1  Table=AeroCoeff.dCY_r_lef
      settings: InputPortMap=u0,u1
  Cy_tot : Outport  VectorParamsAs1DForOutWhenUnconnected=off
  wires:
  Add3/1 -> Product3/1
  beta Prelookup/2 -> CY_delta_r/4, CY_delta_ail_lef/4, CY_delta_ail/4, CY_lef/4, CY/4
  beta Prelookup/1 -> CY_lef/3, CY/3, CY_delta_r/3, CY_delta_ail_lef/3, CY_delta_ail/3
  Product7/1 -> Add4/6
  dlef/1 -> Product6/1, Product4/2, Product/2, Product1/2
  alpha Prelookup/1 -> CY/1, dCY_p_lef/1, CY_p/1, dCY_r_lef/1, CY_r/1, CY_delta_r/1, CY_delta_ail_lef/1, CY_delta_ail/1, CY_lef/1
  Add4/1 -> Cy_tot/1
  Add5/1 -> Product2/1
  CY_p/1 -> Add7/1
  Add1/1 -> Add2/3, Add5/1, [delta_CY_delta_ail]
  CY_lef/1 -> Add2/2, Add/2
  Add/1 -> Product/1
  dCY_p_lef/1 -> Product6/2
  CY_delta_r/1 -> Add3/1
  CY_delta_ail_lef/1 -> Add2/1
  dCY_r_lef/1 -> Product4/1
  alpha (deg)/1 -> alpha Prelookup/1
  CY_r/1 -> Add6/1
  Product4/1 -> Add6/2
  Add2/1 -> Product1/1
  Product3/1 -> Add4/4
  CY/1 -> Add3/2, Add1/1, Add/1, Add4/1
  Product2/1 -> Add4/3
  Product/1 -> Add4/2
  alpha Prelookup/2 -> CY/2, CY_p/2, dCY_p_lef/2, dCY_r_lef/2, CY_r/2, CY_delta_r/2, CY_delta_ail_lef/2, CY_delta_ail/2, CY_lef/2
  Product6/1 -> Add7/2
  Add6/1 -> Product5/2
  Add7/1 -> Product7/1
  Product5/1 -> Add4/5
  Product1/1 -> Add5/2
  CY_delta_ail/1 -> Add1/2
  beta (deg)/1 -> beta Prelookup/1
  Add8/1 -> Gain/1
  drud/1 -> Product3/2
  pb_2v/1 -> Product7/2
  rb_2v/1 -> Product5/1
  right aileron(rad)/1 -> Add8/1
  left aileron(rad)/1 -> Add8/2
  Gain/1 -> Product2/2
  right elevator/1 -> Add9/1
  left elevator/1 -> Add9/2
  [delta_CY_delta_ail] -> Gain2/1
  Add9/1 -> Gain1/1
  Gain1/1 -> Product8/2
  Product8/1 -> Add4/7
  Gain2/1 -> Product8/1

== system Linearization/Vehicle/Aerodynamics/Aerofynamic Coefficients/CZT ==
  note: 氣動力表格僅提供到攻角到
      | 45度，超過45度後皆採用45
      | 度的氣動力係數
  note: ${\hat{Z} }_{\delta_e } =\frac{C_Z {\left(\alpha ,\beta ,\delta_e +0.1\right)}-C_Z {\left(\alpha ,\beta ,\delta_e -0.1\right)}}{0.2}$
  note: $\Delta C_{Z_{LEF} } =C_{Z_{LEF} } {\left(\alpha ,\beta \right)}-C_Z {\left(\alpha ,\beta ,\delta_e =0°\right)}$
  note: $C_{Z,T} =C_Z {\left(\alpha ,\beta ,\delta_e \right)}+\Delta C_{Z_{LEF} } ∙{\left(1-\frac{\delta_{LEF} }{25°}\right)}+\frac{q\overset{-}{c} }{2V_T }∙{\left[C_{Z_q } {\left(\alpha \right)}+\Delta C_{Z_{q_{LEF} } } {\left(\alpha \right)}∙{\left(1-\frac{\delta_{LEF} }{25°}\right)}\right]}+\ \Delta C_{Z_{SB} } {\left(\alpha \right)}∙{\left(\frac{\delta_{SB} }{60°}\right)}+C_{Z_{\delta ra} } \delta_{ra} +C_{Z_{\delta la} } \delta_{la}$
  note: $C_{Z_{\delta ra} } =C_{Z_{\delta la} } =\frac{{\hat{Z} }_{\delta_e } }{2}∙0.4$
  note: 體軸 z 方向之氣動力係數 (total z-axis force coefficient)：
  note: ${\hat{Z} }_{\delta_e } =\frac{C_Z {\left(\alpha ,\beta ,\delta_e +0.1\right)}-C_Z {\left(\alpha ,\beta ,\delta_e -0.1\right)}}{0.2}$
  note: $C_{Z_{\delta ra} } =C_{Z_{\delta la} } =\frac{{\hat{Z} }_{\delta_e } }{2}∙0.4$
  alpha (deg) : Inport
  beta (deg) : Inport  Port=2
  right elevator (deg) : Inport  Port=3
  left elevator (deg) : Inport  Port=4
  dlef : Inport  Port=5
  qc_2v : Inport  Port=6
  sb : Inport  Port=7
  right aileron(rad) : Inport  Port=8
  left aileron(rad) : Inport  Port=9
  Add : Sum  Inputs=+-
  Add1 : Sum  Inputs=+++++
  Add{2..4,7} (4 alike) : Sum
  Add5 : Sum  Inputs=+-
  Add6 : Sum  Inputs=+-
  CZ : Interpolation_n-D  NumberOfTableDimensions=3  Table=AeroCoeff.CZ
      settings: InputPortMap=u0,u1,u2,u3,u4,u5
  CZ1 : Interpolation_n-D  NumberOfTableDimensions=3  Table=AeroCoeff.CZ
      settings: InputPortMap=u0,u1,u2,u3,u4,u5
  CZ2 : Interpolation_n-D  NumberOfTableDimensions=3  Table=AeroCoeff.CZ
      settings: InputPortMap=u0,u1,u2,u3,u4,u5
  CZ_elevator0 : Interpolation_n-D  Table=AeroCoeff.CZ_elevator0
  CZ_lef : Interpolation_n-D  Table=AeroCoeff.CZ_lef
  CZ_q : Interpolation_n-D  NumberOfTableDimensions=1  Table=AeroCoeff.CZ_q
      settings: InputPortMap=u0,u1
  Constant : Constant  Value=0.1
  Constant1 : Constant  Value=0.1
  Constant2 : Constant  Value=0.2
  Divide : Product  Inputs=*/
  Gain : Gain  Gain=20
  Gain2 : Gain  Gain=(1/2)*0.4
  Gain3 : Gain  Gain=20
  Gain4 : Gain  Gain=1/2
  Product{,1..5} (6 alike) : Product
  alpha Prelookup : PreLookup  BreakpointsData=AeroCoeff.alpha_prelookup  IndexSearchMethod=Linear search  BeginIndexSearchUsingPreviousIndexResult=on  DiagnosticForOutOfRangeInput=Warning
  beta Prelookup : PreLookup  BreakpointsData=AeroCoeff.beta_prelookup  IndexSearchMethod=Linear search  BeginIndexSearchUsingPreviousIndexResult=on  DiagnosticForOutOfRangeInput=Warning
  dCZ_q_lef : Interpolation_n-D  NumberOfTableDimensions=1  Table=AeroCoeff.dCZ_q_lef
      settings: InputPortMap=u0,u1
  dCZ_sb : Interpolation_n-D  NumberOfTableDimensions=1  Table=AeroCoeff.dCZ_sb
      settings: InputPortMap=u0,u1
  elevator Prelookup : PreLookup  BreakpointsData=AeroCoeff.elevator_prelookup2  IndexSearchMethod=Linear search  BeginIndexSearchUsingPreviousIndexResult=on  DiagnosticForOutOfRangeInput=Warning
  elevator Prelookup1 : PreLookup  BreakpointsData=AeroCoeff.elevator_prelookup2  IndexSearchMethod=Linear search  BeginIndexSearchUsingPreviousIndexResult=on  DiagnosticForOutOfRangeInput=Warning
  elevator Prelookup2 : PreLookup  BreakpointsData=AeroCoeff.elevator_prelookup2  IndexSearchMethod=Linear search  BeginIndexSearchUsingPreviousIndexResult=on  DiagnosticForOutOfRangeInput=Warning
  Cz_tot : Outport  VectorParamsAs1DForOutWhenUnconnected=off
  wires:
  Product2/1 -> Add1/3
  alpha Prelookup/2 -> dCZ_q_lef/2, dCZ_sb/2, CZ2/2, CZ1/2, CZ_q/2, CZ_elevator0/2, CZ_lef/2, CZ/2
  Add1/1 -> Cz_tot/1
  elevator Prelookup/1 -> CZ/5
  CZ_q/1 -> Add2/1
  beta Prelookup/2 -> CZ/4, CZ_lef/4, CZ_elevator0/4, CZ2/4, CZ1/4
  CZ_lef/1 -> Add/1
  dCZ_q_lef/1 -> Product1/1
  Product1/1 -> Add2/2
  Add2/1 -> Product2/1
  CZ_elevator0/1 -> Add/2
  Add/1 -> Product/1
  dlef/1 -> Product1/2, Product/2
  Product/1 -> Add1/2
  CZ/1 -> Add1/1
  beta Prelookup/1 -> CZ/3, CZ_elevator0/3, CZ2/3, CZ1/3, CZ_lef/3
  alpha Prelookup/1 -> dCZ_q_lef/1, CZ1/1, CZ2/1, dCZ_sb/1, CZ_q/1, CZ_elevator0/1, CZ_lef/1, CZ/1
  alpha (deg)/1 -> alpha Prelookup/1
  elevator Prelookup/2 -> CZ/6
  qc_2v/1 -> Product2/2
  beta (deg)/1 -> beta Prelookup/1
  sb/1 -> Product3/2
  dCZ_sb/1 -> Product3/1
  Product3/1 -> Add1/4
  Constant1/1 -> Add5/2
  CZ2/1 -> Add6/2
  Constant/1 -> Add4/2
  Add5/1 -> elevator Prelookup2/1
  Product5/1 -> Add7/2
  Add4/1 -> elevator Prelookup1/1
  left aileron(rad)/1 -> Gain3/1
  Divide/1 -> Gain2/1
  right aileron(rad)/1 -> Gain/1
  Add6/1 -> Divide/1
  Gain2/1 -> Product5/1, Product4/1
  CZ1/1 -> Add6/1
  Product4/1 -> Add7/1
  Add3/1 -> Gain4/1
  right elevator (deg)/1 -> Add3/1
  left elevator (deg)/1 -> Add3/2
  elevator Prelookup1/1 -> CZ1/5
  elevator Prelookup1/2 -> CZ1/6
  elevator Prelookup2/1 -> CZ2/5
  elevator Prelookup2/2 -> CZ2/6
  Constant2/1 -> Divide/2
  Add7/1 -> Add1/5
  Gain/1 -> Product4/2
  Gain3/1 -> Product5/2
  Gain4/1 -> elevator Prelookup/1, Add5/1, Add4/1

== system Linearization/Vehicle/Aerodynamics/Aerofynamic Coefficients/ClT ==
  note: $\Delta C_{l_{\delta_a } }$
  note: $\Delta C_{l_{{\delta_a }_{LEF} } } =C_{l_{{\delta_a =20°}_{LEF} } } {\left(\alpha ,\beta \right)}-C_{l_{LEF} } {\left(\alpha ,\beta \right)}-\Delta C_{l_{\delta_a } }$
  note: $\Delta C_{l_{\delta_r } } =C_{l_{\delta_r =30°} } {\left(\alpha ,\beta \right)}-C_l {\left(\alpha ,\beta ,\delta_e =0°\right)}$
  note: $\Delta C_{l_{\delta_a } } =C_{l_{\delta_a =20°} } {\left(\alpha ,\beta \right)}-C_l {\left(\alpha ,\beta ,\delta_e =0°\right)}$
  note: $\Delta C_{l_{LEF} } =C_{l_{LEF} } {\left(\alpha ,\beta \right)}-C_l {\left(\alpha ,\beta ,\delta_e =0°\right)}$
  note: 側滾氣動力矩係數 (total rolling moment coefficient)：
  note: 氣動力表格僅提供到攻角到
      | 45度，超過45度後皆採用45
      | 度的氣動力係數
  note: 氣動力表格僅提供到攻角到
      | 45度，超過45度後皆採用45
      | 度的氣動力係數
  note: $C_{l,T} \ \ \ =\ \ \ C_l {\left(\alpha ,\beta ,\delta_e \right)}+\Delta C_{l_{LEF} } ∙{\left(1-\frac{\delta_{LEF} }{25°}\right)}+\frac{pb}{2V_T }∙{\left[C_{l_p } {\left(\alpha \right)}+\Delta C_{l_{p_{LEF} } } {\left(\alpha \right)}∙{\left(1-\frac{\delta_{LEF} }{25°}\right)}\right]}+\frac{rb}{2V_T }∙{\left[C_{l_r } {\left(\alpha \right)}+\Delta C_{l_{r_{LEF} } } {\left(\alpha \right)}∙{\left(1-\frac{\delta_{LEF} }{25°}\right)}\right]}+\Delta C_{l_{\beta } } {\left(\alpha \right)}∙\beta +\Delta C_{l_{\delta_r } } ∙{\left(\frac{\delta_r }{30°}\right)}+\frac{{\left[\Delta C_{l_{\delta_a } } +\Delta C_{l_{{\delta_a }_{LEF} } } ∙{\left(1-\frac{\delta_{LEF} }{25°}\right)}\right]}}{2}∙{\left(\frac{\delta_{ra} }{20°}\right)}-\frac{{\left[\Delta C_{l_{\delta_a } } +\Delta C_{l_{{\delta_a }_{LEF} } } ∙{\left(1-\frac{\delta_{LEF} }{25°}\right)}\right]}}{2}∙{\left(\frac{\delta_{la} }{20°}\right)}+C_{l_{\delta re} } ∙{\left(\frac{\delta_{re} }{25°}\right)}-C_{l_{\delta le} } ∙{\left(\frac{\delta_{le} }{25°}\right)}$
  note: $C_{l_{\delta re} } =C_{l_{\delta le} } =\frac{\Delta C_{l_{\delta_a } } }{2}∙0.56$
  note: $\Delta C_{l_{\delta_a } }$
  note: $C_{l_{\delta re} } =C_{l_{\delta le} } =\frac{\Delta C_{l_{\delta_a } } }{2}∙0.56$
  alpha (deg) : Inport
  beta (deg) : Inport  Port=2
  drud : Inport  Port=3
  dlef : Inport  Port=4
  right aileron(rad) : Inport  Port=5
  left aileron(rad) : Inport  Port=6
  rb_2v : Inport  Port=7
  pb_2v : Inport  Port=8
  right elevator : Inport  Port=9
  left elevator : Inport  Port=10
  Add : Sum  Inputs=+-
  Add1 : Sum  Inputs=+-
  Cl : Interpolation_n-D  NumberOfTableDimensions=3  Table=AeroCoeff.Cl
      settings: InputPortMap=u0,u1,u2,u3,u4,u5
  Cl_delta_ail : Interpolation_n-D  Table=AeroCoeff.Cl_delta_ail  InternalRulePriority=Speed
  Cl_delta_ail_lef : Interpolation_n-D  Table=AeroCoeff.Cl_delta_ail_lef  InternalRulePriority=Speed
  Cl_delta_r : Interpolation_n-D  Table=AeroCoeff.Cl_delta_r  InternalRulePriority=Speed
  Cl_elevator0 : Interpolation_n-D  Table=AeroCoeff.Cl_elevator0
  Cl_lef : Interpolation_n-D  Table=AeroCoeff.Cl_lef  InternalRulePriority=Speed
  Cl_p : Interpolation_n-D  NumberOfTableDimensions=1  Table=AeroCoeff.Cl_p  InternalRulePriority=Speed
      settings: InputPortMap=u0,u1
  Cl_r : Interpolation_n-D  NumberOfTableDimensions=1  Table=AeroCoeff.Cl_r  InternalRulePriority=Speed
      settings: InputPortMap=u0,u1
  Gain : Gain  Gain=1/2
  Gain1 : Gain  Gain=1/25
  Gain2 : Gain  Gain=(1/2)*0.56
  Product{,1..9} (10 alike) : Product
  Subtract : Sum  Inputs=+-
  Subtract1 : Sum  Inputs=+-
  Subtract2 : Sum  Inputs=+--
  Subtract3 : Sum  Inputs=+-
  Subtract4 : Sum  Inputs=++++++++
  Subtract5 : Sum
  Subtract6 : Sum
  Subtract7 : Sum
  alpha Prelookup : PreLookup  BreakpointsData=AeroCoeff.alpha_prelookup  IndexSearchMethod=Linear search  BeginIndexSearchUsingPreviousIndexResult=on  DiagnosticForOutOfRangeInput=Warning
  beta Prelookup : PreLookup  BreakpointsData=AeroCoeff.beta_prelookup  IndexSearchMethod=Linear search  BeginIndexSearchUsingPreviousIndexResult=on  DiagnosticForOutOfRangeInput=Warning
  dCl_beta : Interpolation_n-D  NumberOfTableDimensions=1  Table=AeroCoeff.dCl_beta  InternalRulePriority=Speed
      settings: InputPortMap=u0,u1
  dCl_p_lef : Interpolation_n-D  NumberOfTableDimensions=1  Table=AeroCoeff.dCl_p_lef  InternalRulePriority=Speed
      settings: InputPortMap=u0,u1
  dCl_r_lef : Interpolation_n-D  NumberOfTableDimensions=1  Table=AeroCoeff.dCl_r_lef  InternalRulePriority=Speed
      settings: InputPortMap=u0,u1
  elevator Prelookup : PreLookup  BreakpointsData=AeroCoeff.elevator_prelookup1  IndexSearchMethod=Linear search  BeginIndexSearchUsingPreviousIndexResult=on  DiagnosticForOutOfRangeInput=Warning
  Cl_tot : Outport  VectorParamsAs1DForOutWhenUnconnected=off
  wires:
  Cl_elevator0/1 -> Subtract3/2, Subtract1/2, Subtract/2
  beta Prelookup/1 -> Cl/3, Cl_lef/3, Cl_elevator0/3, Cl_delta_r/3, Cl_delta_ail_lef/3, Cl_delta_ail/3
  Cl_delta_r/1 -> Subtract3/1
  Cl_lef/1 -> Subtract2/3, Subtract/1
  Subtract/1 -> Product/1
  Product6/1 -> Subtract7/2
  alpha Prelookup/1 -> Cl/1, Cl_lef/1, dCl_r_lef/1, dCl_p_lef/1, dCl_beta/1, Cl_p/1, Cl_r/1, Cl_delta_r/1, Cl_delta_ail_lef/1, Cl_delta_ail/1, Cl_elevator0/1
  Product2/1 -> Subtract4/3
  Cl_p/1 -> Subtract7/1
  beta (deg)/1 -> Product8/2, beta Prelookup/1
  Subtract2/1 -> Product1/1
  alpha Prelookup/2 -> Cl/2, Cl_lef/2, Cl_r/2, dCl_r_lef/2, dCl_p_lef/2, dCl_beta/2, Cl_p/2, Cl_delta_r/2, Cl_delta_ail_lef/2, Cl_delta_ail/2, Cl_elevator0/2
  alpha (deg)/1 -> alpha Prelookup/1
  Product/1 -> Subtract4/2
  Subtract6/1 -> Product5/2
  rb_2v/1 -> Product5/1
  Cl_delta_ail/1 -> Subtract1/1
  Subtract5/1 -> Product2/1
  drud/1 -> Product3/2
  elevator Prelookup/1 -> Cl/5
  Product7/1 -> Subtract4/6
  Subtract7/1 -> Product7/1
  Product5/1 -> Subtract4/5
  dCl_r_lef/1 -> Product4/1
  Subtract3/1 -> Product3/1
  Subtract1/1 -> Subtract2/2, Subtract5/1, [delta_Cl_delta_ail]
  dlef/1 -> Product6/1, Product4/2, Product/2, Product1/2
  Product3/1 -> Subtract4/4
  Cl_delta_ail_lef/1 -> Subtract2/1
  beta Prelookup/2 -> Cl/4, Cl_lef/4, Cl_elevator0/4, Cl_delta_ail/4, Cl_delta_r/4, Cl_delta_ail_lef/4
  Product4/1 -> Subtract6/2
  dCl_beta/1 -> Product8/1
  Product1/1 -> Subtract5/2
  dCl_p_lef/1 -> Product6/2
  Product8/1 -> Subtract4/7
  Cl_r/1 -> Subtract6/1
  elevator Prelookup/2 -> Cl/6
  Cl/1 -> Subtract4/1
  Subtract4/1 -> Cl_tot/1
  pb_2v/1 -> Product7/2
  right aileron(rad)/1 -> Add/1
  left aileron(rad)/1 -> Add/2
  Add/1 -> Gain/1
  Gain/1 -> Product2/2
  right elevator/1 -> Add1/1
  left elevator/1 -> Add1/2
  Add1/1 -> Gain1/1, elevator Prelookup/1
  Gain1/1 -> Product9/2
  [delta_Cl_delta_ail] -> Gain2/1
  Gain2/1 -> Product9/1
  Product9/1 -> Subtract4/8
